simulink model "path_following"  (R2016b)
settings: Solver=VariableStepAuto  StartTime=0.0  StopTime=inf  FixedStep=0.01  RelTol=1e-3  EnableMultiTasking=on
undefined symbols (not defined in the file or in its folder): Angular, Linear
libraries: robotlib x3, robotalgslib x1
settings Model: Creator=The MathWorks, Inc.  LastModifiedBy=SangjunLee
settings GRTTargetCC: TargetLangStandard=C89/C90 (ANSI)
settings ConfigComp: CovMetricSettings=dsw  CovHtmlReporting=on  CovSaveCumulativeToWorkspaceVar=on  CovSaveSingleToWorkspaceVar=on  CovExternalEMLEnable=off

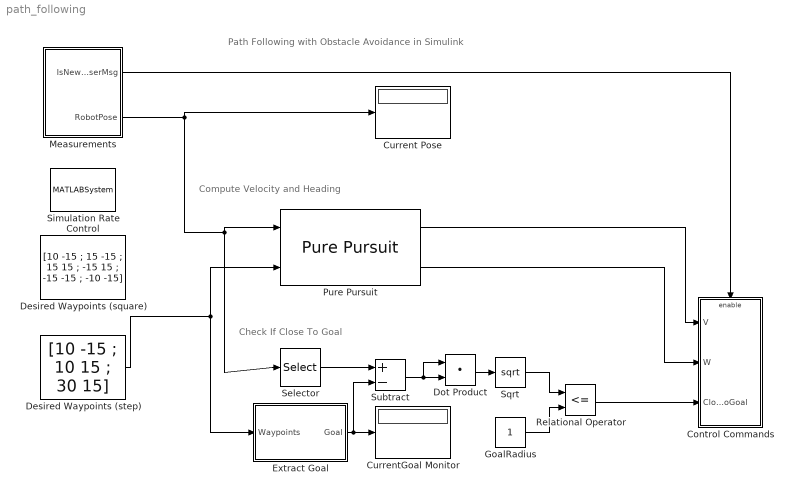
== system path_following ==
  note: Compute Velocity and Heading
  note: Path Following with Obstacle Avoidance in Simulink
  note: Check If Close To Goal
  " Extract Goal" : MATLAB Function  TreatAsAtomicUnit=on
  Control Commands : Subsystem
  Current Pose : Display
  CurrentGoal Monitor : Display
  Desired Waypoints (square) : Constant  Value=[10 -15 ; 15 -15 ; 15 15 ; -15 15 ; -15 -15 ; -10 -15]  OutDataTypeStr=double
  Desired Waypoints (step) : Constant  Value=[10 -15 ; 10 15 ; 30 15]  OutDataTypeStr=double
  Dot Product : DotProduct  InputSameDT=on  OutDataTypeStr=Inherit: Inherit via internal rule
  GoalRadius : Constant
  Measurements : Subsystem
  Pure Pursuit : robotalgslib/Pure Pursuit  DesiredLinearVelocity=2.0  MaxAngularVelocity=1.0  LookaheadDistance=3.5  TargetDirPort=off  SimulateUsing=Code generation
  Relational Operator : RelationalOperator  Operator=<=  OutDataTypeStr=boolean  RndMeth=Simplest
  Selector : Selector  InputPortWidth=3  IndexOptions=Index vector (dialog)  Indices=[1 2]  OutputSizes=1
  Simulation Rate Control : MATLABSystem  System=ExampleHelperSimulationRateControl  SampleTime=0.02
      mask Type: ExampleHelperSimulationRateControl
      mask Display: disp('Rate Control');
  Sqrt : Sqrt  SaturateOnIntegerOverflow=on
  Subtract : Sum  Inputs=+-
  wires:
  Pure Pursuit/1 -> Control Commands/1(V)
  Measurements/1(IsNewLaserMsg) -> Control Commands/Enable
  Pure Pursuit/2 -> Control Commands/2(W)
  Relational Operator/1 -> Control Commands/3(CloseToGoal)
  Subtract/1 -> Dot Product/1, Dot Product/2
  Sqrt/1 -> Relational Operator/1
  Dot Product/1 -> Sqrt/1
  Selector/1 -> Subtract/1
  GoalRadius/1 -> Relational Operator/2
  Measurements/2(RobotPose) -> Selector/1, Pure Pursuit/1, Current Pose/1
  Desired Waypoints (step)/1 -> Pure Pursuit/2, " Extract Goal"/1(Waypoints)
  " Extract Goal"/1(Goal) -> CurrentGoal Monitor/1, Subtract/2

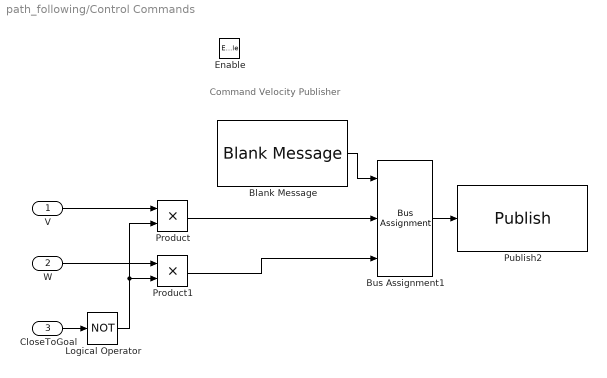
== system path_following/Control Commands ==
  note: Command Velocity Publisher
  V : Inport
  W : Inport  Port=2
  CloseToGoal : Inport  Port=3
  Enable : EnablePort
  Blank Message : robotlib/Blank Message  SourceLibraryInfo=This block requires Robotics System Toolbox  messageType=geometry_msgs/Twist  SampleTime=inf
  Bus Assignment1 : BusAssignment  DialogController=Simulink.DDGSource_BusAssignment  AssignedSignals=Linear.X,Angular.Z
  Logical Operator : Logic  Operator=NOT  AllPortsSameDT=off  OutDataTypeStr=boolean
  Product : Product
  Product1 : Product
  Publish2 : robotlib/Publish  SourceLibraryInfo=This block requires Robotics System Toolbox  topicSource=Select from ROS network  topic=/catvehicle/cmd_vel  messageType=geometry_msgs/Twist  messageQueueLength=105
  wires:
  CloseToGoal/1 -> Logical Operator/1
  V/1 -> Product/1
  W/1 -> Product1/1
  Product1/1 -> Bus Assignment1/3
  Product/1 -> Bus Assignment1/2
  Blank Message/1 -> Bus Assignment1/1
  Bus Assignment1/1 -> Publish2/1
  Logical Operator/1 -> Product1/2, Product/2

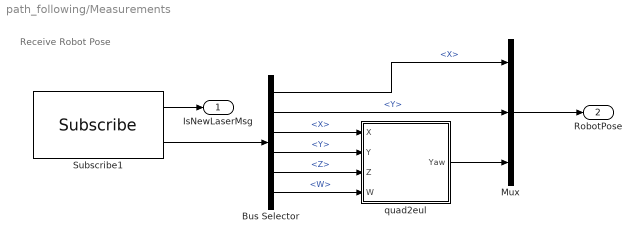
== system path_following/Measurements ==
  note: Receive Robot Pose
  Bus Selector : BusSelector  OutputSignals=Pose.Pose.Position.X,Pose.Pose.Position.Y,Pose.Pose.Orientation.X,Pose.Pose.Orientation.Y,Pose.Pose.Orientation.Z,Pose.Pose.Orientation.W
  Mux : Mux  Inputs=3
  Subscribe1 : robotlib/Subscribe  SourceLibraryInfo=This block requires Robotics System Toolbox  topicSource=Select from ROS network  topic=/catvehicle/odom  messageType=nav_msgs/Odometry  sampleTime=-1  messageQueueLength=1
  quad2eul : MATLAB Function  TreatAsAtomicUnit=on
  IsNewLaserMsg : Outport
  RobotPose : Outport  Port=2
  wires:
  quad2eul/1(Yaw) -> Mux/3
  Subscribe1/2 -> Bus Selector/1
  Bus Selector/3 -> quad2eul/1(X)  "<X>"
  Subscribe1/1 -> IsNewLaserMsg/1
  Bus Selector/2 -> Mux/2  "<Y>"
  Bus Selector/5 -> quad2eul/3(Z)  "<Z>"
  Bus Selector/4 -> quad2eul/2(Y)  "<Y>"
  Bus Selector/1 -> Mux/1  "<X>"
  Bus Selector/6 -> quad2eul/4(W)  "<W>"
  Mux/1 -> RobotPose/1

== matlab function path_following/Measurements/quad2eul ==
  data: X input; Yaw output; Y input; Z input; W input
function Yaw = quat2eulBlk(X, Y, Z, W)
%#codegen

eularAngles = quat2eul([W, X, Y, Z]);
Yaw = eularAngles(1);

== matlab function path_following/ Extract Goal ==
  data: Waypoints input; Goal output
function Goal = extractGoal(Waypoints)
%#codegen
b = isnan(Waypoints);
[rows,~] = find(b);
ridx = setdiff(1:size(Waypoints,1), sort(rows));
Goal = [Waypoints(ridx(end), 1) Waypoints(ridx(end), 2)];
